simulink model "ex6sima"  (R2015a)
settings: Solver=ode45  StartTime=0.0  StopTime=10.0  RelTol=1e-3
values from neighbouring files (symbols this model uses):
  Cden = Cz.den{:}    [runsim.m]
  Cnum = Cz.num{:}    [runsim.m]
  den = Gs.den{1}    [ex6.m]    (also in s2z.m = G.den{1}')
  num = Gs.num{1}    [ex6.m]    (also in s2z.m = G.num{1}')
  Ts = 0.1    [ex3.m]
settings Model: Creator=brunopeixoto  LastModifiedBy=brunopeixoto

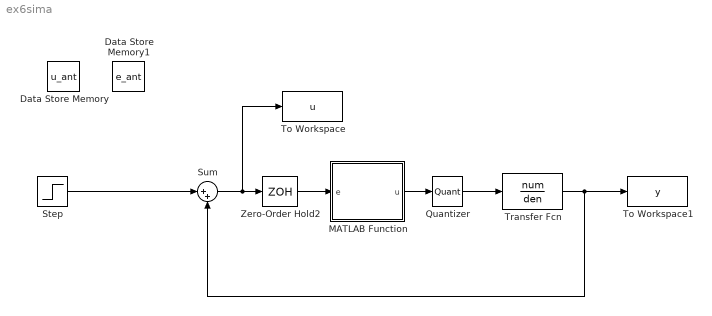
== system ex6sima ==
  Data Store Memory : DataStoreMemory  DataStoreName=u_ant  OutDataTypeStr=double
  Data Store Memory1 : DataStoreMemory  DataStoreName=e_ant  OutDataTypeStr=double
  MATLAB Function : MATLAB Function  TreatAsAtomicUnit=on  SystemSampleTime=Ts
  Quantizer : Quantizer
  Step : Step  SampleTime=0
  Sum : Sum  Inputs=|++
  To Workspace : ToWorkspace  VariableName=u  SaveFormat=Structure With Time  SampleTime=-1
  To Workspace1 : ToWorkspace  VariableName=y  SaveFormat=Structure With Time  SampleTime=-1
  Transfer Fcn : TransferFcn  Numerator=num  Denominator=den
  Zero-Order Hold2 : ZeroOrderHold
  wires:
  MATLAB Function/1(u) -> Quantizer/1
  Quantizer/1 -> Transfer Fcn/1
  Transfer Fcn/1 -> Sum/2, To Workspace1/1
  Step/1 -> Sum/1
  Sum/1 -> To Workspace/1, Zero-Order Hold2/1
  Zero-Order Hold2/1 -> MATLAB Function/1(e)

== matlab function ex6sima/MATLAB Function ==
  settings: updateMethod=DISCRETE  sampleTime=Ts
  data: e input; u output size=1; Cnum parameter; u_ant data_store_memory; Cden parameter; e_ant data_store_memory
function u = fcn(e, Cnum, Cden)
    global u_ant; 
    global e_ant;
    
    m = length(Cnum);
    n = length(Cden);
    
    
    
    a = Cnum;
    b = Cden;

    e_ant(1:end-1) = e_ant(2:end);
    e_ant(end) = e;
    
    u = (b'*e_ant - a(2:end)'*u_ant)/a(1);
    
    assignin('base', 'u', u);
    assignin('base', 'm', m);
    assignin('base', 'n', n);
    
    u_ant(1:end-1) = u_ant(2:end);
    u_ant(end) = u;   
end
